simulink model "break_stand_sim"  (R2021a)
settings: Solver=VariableStepAuto  StartTime=0.0  StopTime=10.0  RelTol=1e-3
undefined symbols (not defined in the file): base_height, base_length, base_mass, extension_height, extension_length, extension_mass, initial_extension, motor_base_height, motor_base_length, motor_base_mass, wheel_mass, wheel_r
settings Model: Creator=Usuario  LastModifiedBy=Usuario

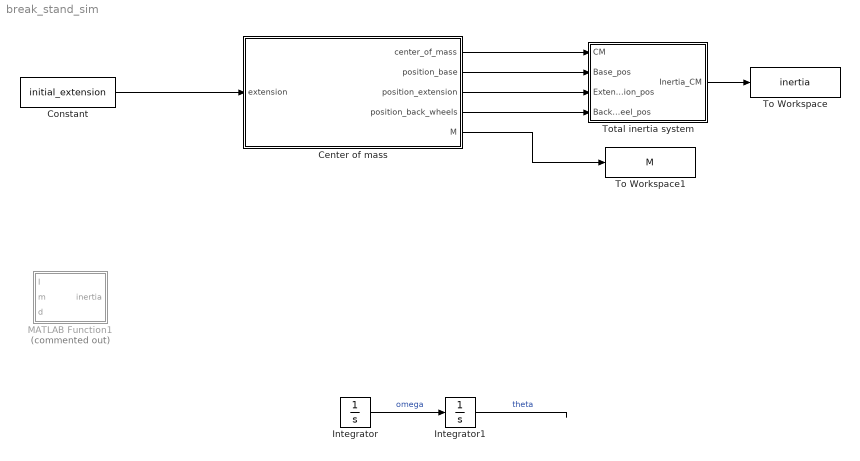
== system break_stand_sim ==
  Center of mass : MATLAB Function  TreatAsAtomicUnit=on
  Constant : Constant  Value=initial_extension
  Integrator : Integrator
  Integrator1 : Integrator
  MATLAB Function1 : MATLAB Function  Commented=on  TreatAsAtomicUnit=on
  To Workspace : ToWorkspace  VariableName=inertia  SaveFormat=Timeseries  SampleTime=-1
  To Workspace1 : ToWorkspace  VariableName=M  SaveFormat=Timeseries  SampleTime=-1
  Total inertia system : Subsystem
  wires:
  Constant/1 -> Center of mass/1(extension)
  Center of mass/1(center_of_mass) -> Total inertia system/1(CM)
  Center of mass/2(position_base) -> Total inertia system/2(Base_pos)
  Center of mass/3(position_extension) -> Total inertia system/3(Extension_pos)
  Center of mass/4(position_back_wheels) -> Total inertia system/4(Back_wheel_pos)
  Total inertia system/1(Inertia_CM) -> To Workspace/1
  Center of mass/5(M) -> To Workspace1/1
  Integrator/1 -> Integrator1/1  "omega"
  ? -> Integrator/1  "alpha"
  Integrator1/1 -> ?  "theta"

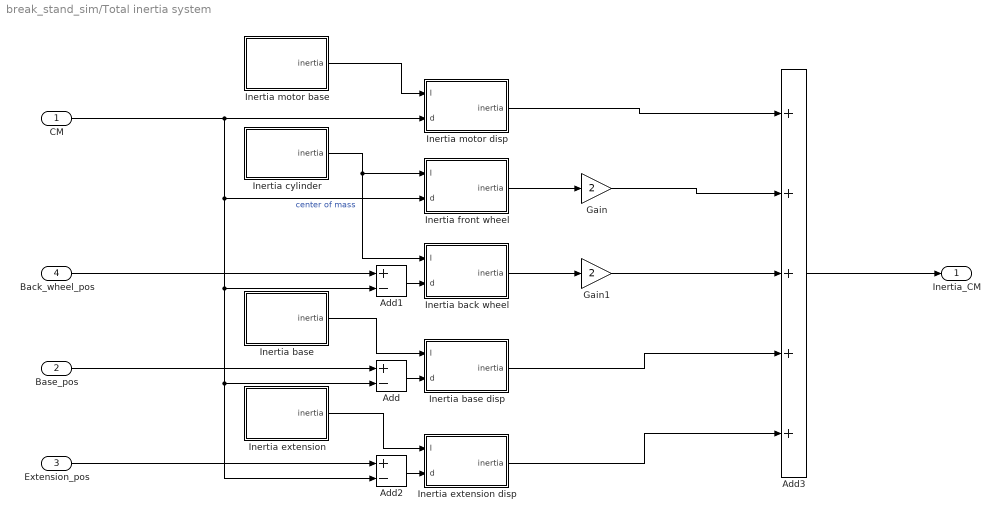
== system break_stand_sim/Total inertia system ==
  CM : Inport
  Base_pos : Inport  Port=2
  Extension_pos : Inport  Port=3
  Back_wheel_pos : Inport  Port=4
  Add : Sum  Inputs=+-
  Add1 : Sum  Inputs=+-
  Add2 : Sum  Inputs=+-
  Add3 : Sum  Inputs=+++++
  Gain : Gain  Gain=2
  Gain1 : Gain  Gain=2
  Inertia back wheel : MATLAB Function  TreatAsAtomicUnit=on
  Inertia base : MATLAB Function  TreatAsAtomicUnit=on
  Inertia base disp : MATLAB Function  TreatAsAtomicUnit=on
  Inertia cylinder : MATLAB Function  TreatAsAtomicUnit=on
  Inertia extension : MATLAB Function  TreatAsAtomicUnit=on
  Inertia extension disp : MATLAB Function  TreatAsAtomicUnit=on
  Inertia front wheel : MATLAB Function  TreatAsAtomicUnit=on
  Inertia motor base : MATLAB Function  TreatAsAtomicUnit=on
  Inertia motor disp : MATLAB Function  TreatAsAtomicUnit=on
  Inertia_CM : Outport
  wires:
  Inertia cylinder/1(inertia) -> Inertia back wheel/1(I), Inertia front wheel/1(I)
  Add1/1 -> Inertia back wheel/2(d)
  Inertia extension/1(inertia) -> Inertia extension disp/1(I)
  Base_pos/1 -> Add/1
  CM/1 -> Add2/2, Add/2, Add1/2, Inertia front wheel/2(d), Inertia motor disp/2(d)  "center of mass"
  Add2/1 -> Inertia extension disp/2(d)
  Inertia base/1(inertia) -> Inertia base disp/1(I)
  Add/1 -> Inertia base disp/2(d)
  Inertia motor base/1(inertia) -> Inertia motor disp/1(I)
  Inertia back wheel/1(inertia) -> Gain1/1
  Inertia front wheel/1(inertia) -> Gain/1
  Extension_pos/1 -> Add2/1
  Back_wheel_pos/1 -> Add1/1
  Add3/1 -> Inertia_CM/1
  Inertia motor disp/1(inertia) -> Add3/1
  Gain/1 -> Add3/2
  Gain1/1 -> Add3/3
  Inertia base disp/1(inertia) -> Add3/4
  Inertia extension disp/1(inertia) -> Add3/5

== matlab function break_stand_sim/Total inertia system/Inertia base disp ==
  data: I input; inertia output; d input; base_mass parameter
function inertia = fcn(I, d, base_mass)
inertia = I + base_mass*d^2;

== matlab function break_stand_sim/Total inertia system/Inertia extension disp ==
  data: I input; inertia output; d input; extension_mass parameter
function inertia = fcn(I, d, extension_mass)
inertia = I + extension_mass*d^2;

== matlab function break_stand_sim/Total inertia system/Inertia cylinder ==
  data: inertia output; wheel_r parameter; wheel_mass parameter
function inertia = fcn(wheel_r, wheel_mass) % cylinder in z
inertia = wheel_mass*wheel_r^2/2;

== matlab function break_stand_sim/Center of mass ==
  data: extension input; center_of_mass output; wheel_mass parameter; base_mass parameter; extension_mass parameter; motor_base_mass parameter; motor_base_length parameter; base_length parameter; position_base output; position_extension output; position_back_wheels output; M output
function [center_of_mass, position_base, position_extension, position_back_wheels, M] = fcn(extension, wheel_mass, base_mass, extension_mass, motor_base_mass, motor_base_length, base_length) % the position of the extension
M = 4*wheel_mass + base_mass + extension_mass + motor_base_mass;
% calculate individual m*r

% position of the motor base
% pos_motor_base = motor_base_length*0.5+base_length*0.5;
% pos_motor_base = 0; % origin

% position of the base
position_base = -(motor_base_length*0.5+base_length*0.5);

% position of the extension
position_extension = -0.1 + extension + position_base;

% position back wheels
position_back_wheels = position_extension - (base_length/2-0.05);

m1 = base_mass * position_base;

% the motor base
% m2 = motor_base_mass * pos_motor_base;
m2 = 0; % origin

% front wheels
% m3 = 2*wheel_mass * pos_motor_base;
m3 = 0; % origin

% extension
m4 = extension_mass * position_extension;

% back wheels
m5 = 2*wheel_mass * position_back_wheels;

% final result
center_of_mass = (m1+m2+m3+m4+m5)/M;

== matlab function break_stand_sim/Total inertia system/Inertia base ==
  data: inertia output; base_height parameter; base_length parameter; base_mass parameter
function inertia = fcn(base_height, base_length, base_mass) % inertia of a box
inertia = base_mass/12*(base_height^2+base_length^2);

== matlab function break_stand_sim/Total inertia system/Inertia extension ==
  data: inertia output; extension_height parameter; extension_length parameter; extension_mass parameter
function inertia = fcn(extension_height, extension_length, extension_mass) % inertia of a box
inertia = extension_mass/12*(extension_height^2+extension_length^2);

== matlab function break_stand_sim/Total inertia system/Inertia motor base ==
  data: inertia output; motor_base_height parameter; motor_base_length parameter; motor_base_mass parameter
function inertia = fcn(motor_base_height, motor_base_length, motor_base_mass) % inertia of a box
inertia = motor_base_mass/12*(motor_base_height^2+motor_base_length^2);

== matlab function break_stand_sim/Total inertia system/Inertia front wheel ==
  data: I input; inertia output; d input; wheel_mass parameter
function inertia = fcn(I, d, wheel_mass)
inertia = I + wheel_mass*d^2;

== matlab function break_stand_sim/MATLAB Function1 ==
  data: I input; inertia output; m input; d input
function inertia = fcn(I, m, d)
inertia = I + m*d^2;

== matlab function break_stand_sim/Total inertia system/Inertia back wheel ==
  data: I input; inertia output; d input; wheel_mass parameter
function inertia = fcn(I, d, wheel_mass)
inertia = I + wheel_mass*d^2;

== matlab function break_stand_sim/Total inertia system/Inertia motor disp ==
  data: I input; inertia output; d input; motor_base_mass parameter
function inertia = fcn(I, d, motor_base_mass)
inertia = I + motor_base_mass*d^2;
